simulink model "PI_controller"  (R2017a)
settings: Solver=VariableStepAuto  StartTime=0.0  StopTime=20  RelTol=1e-3
values from neighbouring files (symbols this model uses):
  Cs_1 = tf([Kc_1*tau_1 Kc_1], [tau_1 0])    [PI_controller_params.m]
  Cs_2 = tf([Kc_2*tau_2 Kc_2], [tau_2 0])    [PI_controller_params.m]
  Gs = tf([-1 0.4],[1 0.5 0.04])    [PID_controller_params.m]    (also in PI_controller_params.m = tf([0.1],[10 1]))
settings Model: Creator=adityaaaap  LastModifiedBy=adityaaaap

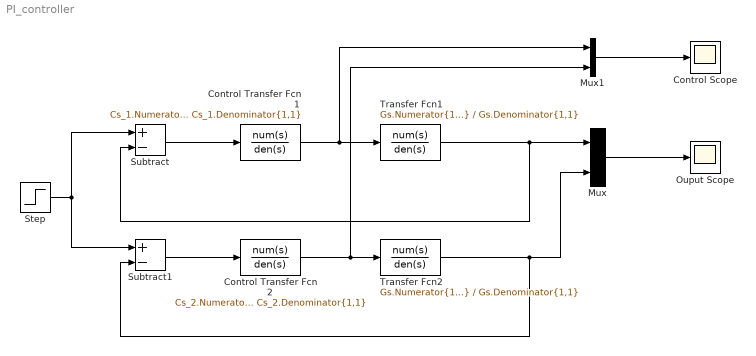
== system PI_controller ==
  "Control Scope " : Scope
  Control Transfer Fcn 1 : TransferFcn  Numerator=Cs_1.Numerator{1,1}  Denominator=Cs_1.Denominator{1,1}
  Control Transfer Fcn 2 : TransferFcn  Numerator=Cs_2.Numerator{1,1}  Denominator=Cs_2.Denominator{1,1}
  Mux : Mux  Inputs=2
  Mux1 : Mux  Inputs=2
  "Ouput Scope " : Scope
  Step : Step  Time=0  SampleTime=0
  Subtract : Sum  Inputs=+-
  Subtract1 : Sum  Inputs=+-
  Transfer Fcn1 : TransferFcn  Numerator=Gs.Numerator{1,1}  Denominator=Gs.Denominator{1,1}
  Transfer Fcn2 : TransferFcn  Numerator=Gs.Numerator{1,1}  Denominator=Gs.Denominator{1,1}
  wires:
  Step/1 -> Subtract/1, Subtract1/1
  Subtract/1 -> Control Transfer Fcn 1/1
  Control Transfer Fcn 1/1 -> Mux1/1, Transfer Fcn1/1
  Transfer Fcn1/1 -> Subtract/2, Mux/1
  Mux/1 -> "Ouput Scope "/1
  Subtract1/1 -> Control Transfer Fcn 2/1
  Control Transfer Fcn 2/1 -> Mux1/2, Transfer Fcn2/1
  Transfer Fcn2/1 -> Mux/2, Subtract1/2
  Mux1/1 -> "Control Scope "/1
